simulink model "VDSE_2019b1"  (R2022b)
settings: Solver=ode5  StartTime=0.0  StopTime=T_simulation  FixedStep=simulation_step_time  RelTol=1e-3
values from neighbouring files (symbols this model uses):
  A = 2    [vehicle_parameters_script.m]
  bump_height = 0    [vehicle_parameters_script.m]
  bump_length = 0    [vehicle_parameters_script.m]
  bump_time = 0    [vehicle_parameters_script.m]
  cd = 0.35    [vehicle_parameters_script.m]
  cF = 5000    [vehicle_parameters_script.m]
  clF = -0.15    [vehicle_parameters_script.m]
  clR = -0.20    (= -0.2)    [vehicle_parameters_script.m]
  cp_FA = 30    [vehicle_parameters_script.m]
  cp_RA = 13    [vehicle_parameters_script.m]
  cR = 5000    [vehicle_parameters_script.m]
  ctF = tireF.VERTICAL_DAMPING    [vehicle_parameters_script.m]
  ctR = tireR.VERTICAL_DAMPING    [vehicle_parameters_script.m]
  enableDriverControl = 1    [vehicle_parameters_script.m]
  enableLongDynamics = 1    [vehicle_parameters_script.m]
  enablePowertrain = 1    [vehicle_parameters_script.m]
  g = 9.806    [vehicle_parameters_script.m]
  Gear_numbers = [1 2 3 4 5 6]    [vehicle_parameters_script.m]
  GR = [2.9 1.8 1.3 1 0.85 0.75]    [vehicle_parameters_script.m]
  hcog = 0.441    [vehicle_parameters_script.m]
  hpc = 0.0    (= 0)    [vehicle_parameters_script.m]
  hrcF = 0.3    [vehicle_parameters_script.m]
  hrcg = (hrcF*lR+hrcR*lF)/(lF+lR)    (= 0.25108)    [vehicle_parameters_script.m]
  hrcR = 0.2    [vehicle_parameters_script.m]
  huFcog = 0.32    [vehicle_parameters_script.m]
  huRcog = 0.32    [vehicle_parameters_script.m]
  i1 = 11.42    [vehicle_parameters_script.m]
  i2 = 3.727    [vehicle_parameters_script.m]
  initial_gear = 1    [vehicle_parameters_script.m]
  JwF = 2.45    [vehicle_parameters_script.m]
  JwR = 2.45    [vehicle_parameters_script.m]
  Jx = 4.12    [vehicle_parameters_script.m]
  Jy = 109.16    [vehicle_parameters_script.m]
  Jz = 105.13    [vehicle_parameters_script.m]
  kF = 40000    [vehicle_parameters_script.m]
  kR = 35000    [vehicle_parameters_script.m]
  kRF = 0    [vehicle_parameters_script.m]
  kRR = 0    [vehicle_parameters_script.m]
  ktF = tireF.VERTICAL_STIFFNESS    [vehicle_parameters_script.m]
  ktR = tireR.VERTICAL_STIFFNESS    [vehicle_parameters_script.m]
  lF = 1.223    [vehicle_parameters_script.m]
  lR = l-lF    (= 1.277)    [vehicle_parameters_script.m]
  m = 340    [vehicle_parameters_script.m]
  max_pressure = 1000    [vehicle_parameters_script.m]
  maxrpm = 4000    [vehicle_parameters_script.m]
  mF = 45    [vehicle_parameters_script.m]
  minrpm = 1500    [vehicle_parameters_script.m]
  mR = 50    [vehicle_parameters_script.m]
  output_samping_time = 0.001    [vehicle_parameters_script.m]
  phi0 = 0    [vehicle_parameters_script.m]
  phi_dot0 = 0    [vehicle_parameters_script.m]
  psi0 = 0    [vehicle_parameters_script.m]
  psi_dot0 = 0    [vehicle_parameters_script.m]
  RearRatio = 1    [vehicle_parameters_script.m]
  requested_speed = 120/3.6    (= 33.3333333333)    [vehicle_parameters_script.m]
  rF = tireF.UNLOADED_RADIUS    [vehicle_parameters_script.m]
  rho = 1.2    [vehicle_parameters_script.m]
  rR = tireR.UNLOADED_RADIUS    [vehicle_parameters_script.m]
  steer_ratio = 13.25    [vehicle_parameters_script.m]
  TFL = 0    [vehicle_parameters_script.m]
  TFR = 0    [vehicle_parameters_script.m]
  theta0 = 0    [vehicle_parameters_script.m]
  theta_dot0 = 0    [vehicle_parameters_script.m]
  TRL = 0    [vehicle_parameters_script.m]
  TRR = 0    [vehicle_parameters_script.m]
  Vx0 = 0.01/3.6    (= 0.00277777777778)    [vehicle_parameters_script.m]
  Vy0 = 0    [vehicle_parameters_script.m]
  Vz0 = 0    [vehicle_parameters_script.m]
  wF = 1.578    [vehicle_parameters_script.m]
  wR = 1.544    [vehicle_parameters_script.m]
  x0 = 0    [vehicle_parameters_script.m]
  xcog_overall = (2*mR*xR+2*xF*mF+m*xs)/(m+2*mF+2*mR)    (= 1.25626415094)    [vehicle_parameters_script.m]
  y0 = 0    [vehicle_parameters_script.m]
  z0 = 0    [vehicle_parameters_script.m]
  zFL0 = 0    [vehicle_parameters_script.m]
  zFL_dot0 = 0    [vehicle_parameters_script.m]
  zFR0 = 0    [vehicle_parameters_script.m]
  zFR_dot0 = 0    [vehicle_parameters_script.m]
  zRL0 = 0    [vehicle_parameters_script.m]
  zRL_dot0 = 0    [vehicle_parameters_script.m]
  zRR0 = 0    [vehicle_parameters_script.m]
  zRR_dot0 = 0    [vehicle_parameters_script.m]
undefined symbols (not defined in the file or in its folder): Bxf, Bxr, Byf, Byr, Cxf, Cxr, Cyf, Cyr, DiscIntNeverNeededParam, Dxf, Dxr, Dyf, Dyr, exf, exr, eyf, eyr, FNOMINf, FNOMINr, Ldwf, Ldwr, PCX1f, PCX1r, PCY1f, PCY1r, PDX1f, PDX1r, PDX2f, PDX2r, PDY1f, PDY1r, PDY2f, PDY2r, PDY3f, PDY3r, PEX1f, PEX1r, PEX2f, PEX2r, PEX3f, PEX3r, PEX4f, PEX4r, PEY1f, PEY1r, PEY2f, PEY2r, PEY3f, PEY3r, PEY4f, PEY4r, PHX1f, PHX1r, PHX2f, PHX2r, PHY1f, PHY1r, PHY2f, PHY2r, PHY3f ... (+147)
libraries: simulink x55, mfeval_LIB x4, slpidlib x1
(part 3 of 7)

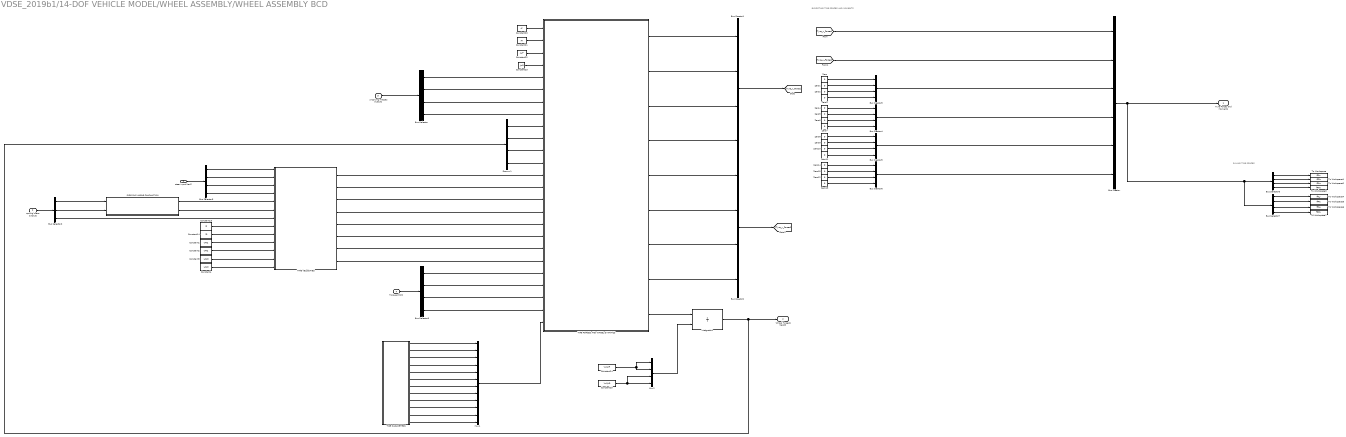
== system VDSE_2019b1/14-DOF VEHICLE MODEL/WHEEL ASSEMBLY/WHEEL ASSEMBLY BCD ==
  note: EXPORTING TIRE FORCES AND MOMENTS
  note: SAVING TIRE FORCES
  steer input [rad] : Inport
  sprung mass outputs : Inport  Port=2
  unsprung masses outputs : Inport  Port=3
  Torques [Nm] : Inport  Port=4
  Bus Creator : BusCreator  Inputs=6
  Bus Creator{1..6} (6 alike) : BusCreator  Inputs=4
  Bus Selector : BusSelector  OutputSignals=Unsprung masses z Forces [N].FLz_Overall [N],Unsprung masses z Forces [N].FRz_Overall [N],Unsprung masses z Forces [N].RLz_Overall [N],Unsprung masses z Forces [N].RRz_Overall [N]
  Bus Selector2 : BusSelector  OutputSignals=Longitudinal Dynamics.Vx [m/s],Lateral Dynamics.Vy [m/s],Yaw dynamics.psi_dot [rad/s]
  Bus Selector3 : BusSelector  OutputSignals=Steering.deltaFL [rad],Steering.deltaFR [rad],Steering.deltaRL [rad],Steering.deltaRR [rad]
  Bus Selector5 : BusSelector  OutputSignals=TFL [Nm],TFR [Nm],TRL [Nm],TRR [Nm]
  Bus Selector6 : BusSelector  OutputSignals=Tyre x Forces [N].fFLx [N],Tyre x Forces [N].fFRx [N],Tyre x Forces [N].fRLx [N],Tyre x Forces [N].fRRx [N]
  Bus Selector7 : BusSelector  OutputSignals=Tyre y Forces [N].fFLy [N],Tyre y Forces [N].fFRy [N],Tyre y Forces [N].fRLy [N],Tyre y Forces [N].fRRy [N]
  Constant1 : Constant  Value=wF/2
  Constant13 : Constant  Value=lF
  Constant14 : Constant  Value=lR
  Constant2 : Constant  Value=wF/2
  Constant20 : Constant  Value=rF
  Constant21 : Constant  Value=rR
  Constant22 : Constant  Value=JwF
  Constant23 : Constant  Value=JwR
  Constant24 : Constant  Value=Vx0/rF
  Constant25 : Constant  Value=Vx0/rR
  Constant3 : Constant  Value=wR/2
  Constant4 : Constant  Value=wR/2
  Demux1 : Demux
  Integrator1 : Integrator  InitialConditionSource=external
  Mux1 : Mux  Inputs=12
  Mux2 : Mux
  SIDE SLIP ANGLE CALCULATION : Subsystem
  TIRE FORCES AND WHEEL DYNAMICS : MATLAB Function  TreatAsAtomicUnit=on
  TIRE PARAMETERS : Subsystem
  TIRE VELOCITIES : MATLAB Function  TreatAsAtomicUnit=on
  To Workspace : ToWorkspace  VariableName=fFLx  SaveFormat=Timeseries  SampleTime=-1
  To Workspace1 : ToWorkspace  VariableName=fFRx  SaveFormat=Timeseries  SampleTime=-1
  To Workspace2 : ToWorkspace  VariableName=fRLx  SaveFormat=Timeseries  SampleTime=-1
  To Workspace3 : ToWorkspace  VariableName=fRRx  SaveFormat=Timeseries  SampleTime=-1
  To Workspace4 : ToWorkspace  VariableName=fFLy  SaveFormat=Timeseries  SampleTime=-1
  To Workspace5 : ToWorkspace  VariableName=fFRy  SaveFormat=Timeseries  SampleTime=-1
  To Workspace6 : ToWorkspace  VariableName=fRLy  SaveFormat=Timeseries  SampleTime=-1
  To Workspace7 : ToWorkspace  VariableName=fRRy  SaveFormat=Timeseries  SampleTime=-1
  Zero{,1..15} (16 alike) : Constant  Value=0  OutDataTypeStr=Inherit: Inherit via back propagation
  Tyre Forces and Moments : Outport
  Wheel Speeds [rad/s] : Outport  Port=2
  wires:
  Bus Selector7/4 -> To Workspace7/1  "<fRRy [N]>"
  Bus Selector7/3 -> To Workspace6/1  "<fRLy [N]>"
  Bus Selector7/2 -> To Workspace5/1  "<fFRy [N]>"
  Bus Selector7/1 -> To Workspace4/1  "<fFLy [N]>"
  Bus Selector6/4 -> To Workspace3/1  "<fRRx [N]>"
  Bus Selector6/3 -> To Workspace2/1  "<fRLx [N]>"
  Bus Selector6/2 -> To Workspace1/1  "<fFRx [N]>"
  Bus Selector6/1 -> To Workspace/1  "<fFLx [N]>"
  Torques [Nm]/1 -> Bus Selector5/1
  Bus Creator/1 -> Tyre Forces and Moments/1, Bus Selector6/1, Bus Selector7/1
  steer input [rad]/1 -> Bus Selector3/1
  Bus Selector3/3 -> TIRE VELOCITIES/3(deltaRL)  "<deltaRL [rad]>"
  Bus Selector3/1 -> TIRE VELOCITIES/1(deltaFL)  "<deltaFL [rad]>"
  Bus Selector3/4 -> TIRE VELOCITIES/4(deltaRR)  "<deltaRR [rad]>"
  Bus Selector3/2 -> TIRE VELOCITIES/2(deltaFR)  "<deltaFR [rad]>"
  sprung mass outputs/1 -> Bus Selector2/1
  Bus Selector2/3 -> TIRE VELOCITIES/7(psidot)  "<psi_dot [rad/s]>"
  Bus Selector2/2 -> SIDE SLIP ANGLE CALCULATION/2(Vy [m/s])  "<Vy [m/s]>"
  Bus Selector2/1 -> SIDE SLIP ANGLE CALCULATION/1(Vx [m/s])  "<Vx [m/s]>"
  unsprung masses outputs/1 -> Bus Selector/1
  Bus Selector/2 -> TIRE FORCES AND WHEEL DYNAMICS/6(fFRz)  "<FRz_Overall [N]>"
  Bus Selector/3 -> TIRE FORCES AND WHEEL DYNAMICS/7(fRLz)  "<RLz_Overall [N]>"
  Bus Selector/4 -> TIRE FORCES AND WHEEL DYNAMICS/8(fRRz)  "<RRz_Overall [N]>"
  Bus Selector/1 -> TIRE FORCES AND WHEEL DYNAMICS/5(fFLz)  "<FLz_Overall [N]>"
  SIDE SLIP ANGLE CALCULATION/1(V [m/s]) -> TIRE VELOCITIES/5(V)  "V"
  SIDE SLIP ANGLE CALCULATION/2(beta [rad]) -> TIRE VELOCITIES/6(beta)  "beta"
  TIRE VELOCITIES/6(VRLy) -> TIRE FORCES AND WHEEL DYNAMICS/18(VRLy)  "VRLy"
  TIRE VELOCITIES/3(VFRx) -> TIRE FORCES AND WHEEL DYNAMICS/15(VFRx)  "VFRx"
  Constant3/1 -> TIRE VELOCITIES/12(wRL)
  TIRE VELOCITIES/5(VRLx) -> TIRE FORCES AND WHEEL DYNAMICS/17(VRLx)  "VRLx"
  Constant2/1 -> TIRE VELOCITIES/11(wFR)
  Constant14/1 -> TIRE VELOCITIES/9(lR)
  Constant1/1 -> TIRE VELOCITIES/10(wFL)
  Constant13/1 -> TIRE VELOCITIES/8(lF)
  Constant4/1 -> TIRE VELOCITIES/13(wRR)
  TIRE VELOCITIES/4(VFRy) -> TIRE FORCES AND WHEEL DYNAMICS/16(VFRy)  "VFRy"
  TIRE VELOCITIES/1(VFLx) -> TIRE FORCES AND WHEEL DYNAMICS/13(VFLx)  "VFLx"
  TIRE VELOCITIES/2(VFLy) -> TIRE FORCES AND WHEEL DYNAMICS/14(VFLy)  "VFLy"
  TIRE PARAMETERS/7(Byf) -> Mux1/7
  TIRE PARAMETERS/6(Dxr) -> Mux1/6
  TIRE PARAMETERS/12(Dyr) -> Mux1/12
  TIRE PARAMETERS/2(Cxf) -> Mux1/2
  Mux1/1 -> TIRE FORCES AND WHEEL DYNAMICS/25(TireParams)
  TIRE PARAMETERS/8(Cyf) -> Mux1/8
  TIRE PARAMETERS/9(Dyf) -> Mux1/9
  TIRE PARAMETERS/5(Cxr) -> Mux1/5
  TIRE PARAMETERS/3(Dxf) -> Mux1/3
  TIRE PARAMETERS/11(Cyr) -> Mux1/11
  TIRE PARAMETERS/10(Byr) -> Mux1/10
  TIRE PARAMETERS/4(Bxr) -> Mux1/4
  TIRE PARAMETERS/1(Bxf) -> Mux1/1
  Constant20/1 -> TIRE FORCES AND WHEEL DYNAMICS/1(rF)
  Constant22/1 -> TIRE FORCES AND WHEEL DYNAMICS/3(JwF)
  Constant23/1 -> TIRE FORCES AND WHEEL DYNAMICS/4(JwR)
  Constant21/1 -> TIRE FORCES AND WHEEL DYNAMICS/2(rR)
  Constant24/1 -> Mux2/2, Mux2/1
  Mux2/1 -> Integrator1/2
  Constant25/1 -> Mux2/3, Mux2/4
  TIRE FORCES AND WHEEL DYNAMICS/9(omega_dot) -> Integrator1/1  "omegas_dot [rad/s^2]"
  Demux1/1 -> TIRE FORCES AND WHEEL DYNAMICS/9(omegaFL)
  Demux1/2 -> TIRE FORCES AND WHEEL DYNAMICS/10(omegaFR)
  Demux1/3 -> TIRE FORCES AND WHEEL DYNAMICS/11(omegaRL)
  Demux1/4 -> TIRE FORCES AND WHEEL DYNAMICS/12(omegaRR)
  Integrator1/1 -> Demux1/1, Wheel Speeds [rad/s]/1  "omega [rad/s]"
  TIRE VELOCITIES/7(VRRx) -> TIRE FORCES AND WHEEL DYNAMICS/19(VRRx)  "VRRx"
  TIRE VELOCITIES/8(VRRy) -> TIRE FORCES AND WHEEL DYNAMICS/20(VRRy)  "VRRy"
  TIRE FORCES AND WHEEL DYNAMICS/6(fFRy) -> Bus Creator2/2  "fFRy [N]"
  TIRE FORCES AND WHEEL DYNAMICS/3(fRLx) -> Bus Creator1/3  "fRLx [N]"
  TIRE FORCES AND WHEEL DYNAMICS/4(fRRx) -> Bus Creator1/4  "fRRx [N]"
  Bus Creator1/1 -> [Tyre_x_Forces]  "Tyre x Forces [N]"
  TIRE FORCES AND WHEEL DYNAMICS/5(fFLy) -> Bus Creator2/1  "fFLy [N]"
  TIRE FORCES AND WHEEL DYNAMICS/7(fRLy) -> Bus Creator2/3  "fRLy [N]"
  TIRE FORCES AND WHEEL DYNAMICS/8(fRRy) -> Bus Creator2/4  "fRRy [N]"
  Bus Creator2/1 -> [Tyre_y_Forces]  "Tyre y Forces [N]"
  Zero6/1 -> Bus Creator4/3  "mRLx [Nm]"
  Zero3/1 -> Bus Creator3/4  "fRRz [N]"
  Zero5/1 -> Bus Creator4/2  "mFRx [Nm]"
  Zero7/1 -> Bus Creator4/4  "mRRx [Nm]"
  Zero1/1 -> Bus Creator3/2  "fFRz [N]"
  Zero4/1 -> Bus Creator4/1  "mFLx [Nm]"
  Zero2/1 -> Bus Creator3/3  "fRLz [N]"
  Zero/1 -> Bus Creator3/1  "fFLz [N]"
  Zero13/1 -> Bus Creator6/4  "mRRz [Nm]"
  Zero12/1 -> Bus Creator6/3  "mRLz [Nm]"
  Zero15/1 -> Bus Creator6/2  "mFRz [Nm]"
  Zero14/1 -> Bus Creator6/1  "mFLz [Nm]"
  TIRE FORCES AND WHEEL DYNAMICS/1(fFLx) -> Bus Creator1/1  "fFLx [N]"
  TIRE FORCES AND WHEEL DYNAMICS/2(fFRx) -> Bus Creator1/2  "fFRx [N]"
  [Tyre_x_Forces] -> Bus Creator/1  "Tyre x Forces [N]"
  [Tyre_y_Forces] -> Bus Creator/2  "Tyre y Forces [N]"
  Bus Creator3/1 -> Bus Creator/3  "Tyre z Forces [N]"
  Bus Creator4/1 -> Bus Creator/4  "Tyre Mx Moments [Nm]"
  Bus Creator5/1 -> Bus Creator/5  "Tyre My Moments [Nm]"
  Bus Creator6/1 -> Bus Creator/6  "Tyre Mz Moments [Nm]"
  Zero8/1 -> Bus Creator5/1  "mFLy [Nm]"
  Zero9/1 -> Bus Creator5/2  "mFRy [Nm]"
  Zero10/1 -> Bus Creator5/3  "mRLy [Nm]"
  Zero11/1 -> Bus Creator5/4  "mRRy [Nm]"
  Bus Selector5/1 -> TIRE FORCES AND WHEEL DYNAMICS/21(TFL)  "<TFL [Nm]>"
  Bus Selector5/2 -> TIRE FORCES AND WHEEL DYNAMICS/22(TFR)  "<TFR [Nm]>"
  Bus Selector5/3 -> TIRE FORCES AND WHEEL DYNAMICS/23(TRL)  "<TRL [Nm]>"
  Bus Selector5/4 -> TIRE FORCES AND WHEEL DYNAMICS/24(TRR)  "<TRR [Nm]>"

== system VDSE_2019b1/14-DOF VEHICLE MODEL/WHEEL ASSEMBLY/WHEEL ASSEMBLY MFEVAL ==
  note: EXPORT TIRE FORCES AND MOMENTS
  note: Wheel Dynamics:
      |
      | J_w∙ω_FR_dot=T_FR- F_FR∙r_w
      | J_w∙ω_FL_dot=T_FL- F_FL∙r_w
      | J_w∙ω_RL_dot= T_RL- F_RL∙r_w
      | J_w∙ω_RR_dot= T_RR- F_RR∙r_w
  note: SAVING TIRE FORCES
  steer input [rad] : Inport
  sprung mass outputs : Inport  Port=2
  unsprung masses outputs : Inport  Port=3
  Torques [Nm] : Inport  Port=4
  Bus Creator : BusCreator  Inputs=6
  Bus Selector : BusSelector  OutputSignals=Unsprung masses z Forces [N].FLz_Overall [N],Unsprung masses z Forces [N].FRz_Overall [N],Unsprung masses z Forces [N].RLz_Overall [N],Unsprung masses z Forces [N].RRz_Overall [N]
  Bus Selector1 : BusSelector  OutputSignals=fFLx [N],fFRx [N],fRLx [N],fRRx [N]
  Bus Selector2 : BusSelector  OutputSignals=Longitudinal Dynamics.Vx [m/s],Lateral Dynamics.Vy [m/s],Yaw dynamics.psi_dot [rad/s]
  Bus Selector3 : BusSelector  OutputSignals=Steering.deltaFL [rad],Steering.deltaFR [rad],Steering.deltaRL [rad],Steering.deltaRR [rad]
  Bus Selector5 : BusSelector  OutputSignals=TFL [Nm],TFR [Nm],TRL [Nm],TRR [Nm]
  Bus Selector6 : BusSelector  OutputSignals=Tyre x Forces [N].fFLx [N],Tyre x Forces [N].fFRx [N],Tyre x Forces [N].fRLx [N],Tyre x Forces [N].fRRx [N]
  Bus Selector7 : BusSelector  OutputSignals=Tyre y Forces [N].fFLy [N],Tyre y Forces [N].fFRy [N],Tyre y Forces [N].fRLy [N],Tyre y Forces [N].fRRy [N]
  Constant : Constant  Value=Vx0/rF
  Constant1 : Constant  Value=wF/2
  Constant13 : Constant  Value=lF
  Constant14 : Constant  Value=lR
  Constant2 : Constant  Value=wF/2
  Constant3 : Constant  Value=wR/2
  Constant4 : Constant  Value=wR/2
  Constant5 : Constant  Value=rF
  Constant6 : Constant  Value=rR
  Constant7 : Constant  Value=Vx0/rR
  Constant8 : Constant  Value=JwF
  Constant9 : Constant  Value=JwR
  Demux : Demux
  Integrator2 : Integrator  InitialConditionSource=external
  Mux : Mux
  SIDE SLIP ANGLE CALCULATION : Subsystem
  Saturation : Saturate  UpperLimit=5000  LowerLimit=-5000
  TIRE CALCULATION : Subsystem
  TIRE VELOCITIES : MATLAB Function  TreatAsAtomicUnit=on
  To Workspace : ToWorkspace  VariableName=fFLx  SaveFormat=Timeseries  SampleTime=-1
  To Workspace1 : ToWorkspace  VariableName=fFRx  SaveFormat=Timeseries  SampleTime=-1
  To Workspace2 : ToWorkspace  VariableName=fRLx  SaveFormat=Timeseries  SampleTime=-1
  To Workspace3 : ToWorkspace  VariableName=fRRx  SaveFormat=Timeseries  SampleTime=-1
  To Workspace4 : ToWorkspace  VariableName=fFLy  SaveFormat=Timeseries  SampleTime=-1
  To Workspace5 : ToWorkspace  VariableName=fFRy  SaveFormat=Timeseries  SampleTime=-1
  To Workspace6 : ToWorkspace  VariableName=fRLy  SaveFormat=Timeseries  SampleTime=-1
  To Workspace7 : ToWorkspace  VariableName=fRRy  SaveFormat=Timeseries  SampleTime=-1
  WHEEL DYNAMICS : MATLAB Function  TreatAsAtomicUnit=on
  Tyre Forces and Moments : Outport
  Wheel Speeds [rad/s] : Outport  Port=2
  wires:
  TIRE CALCULATION/4(Tyre Mx Moments [Nm]) -> Bus Creator/4  "Tyre Mx Moments [Nm]"
  Bus Selector7/4 -> To Workspace7/1  "<fRRy [N]>"
  Bus Selector7/3 -> To Workspace6/1  "<fRLy [N]>"
  Bus Selector7/2 -> To Workspace5/1  "<fFRy [N]>"
  Bus Selector7/1 -> To Workspace4/1  "<fFLy [N]>"
  Bus Selector6/4 -> To Workspace3/1  "<fRRx [N]>"
  Bus Selector6/3 -> To Workspace2/1  "<fRLx [N]>"
  Bus Selector6/2 -> To Workspace1/1  "<fFRx [N]>"
  Bus Selector6/1 -> To Workspace/1  "<fFLx [N]>"
  Torques [Nm]/1 -> Bus Selector5/1
  Bus Creator/1 -> Bus Selector6/1, Bus Selector7/1, Tyre Forces and Moments/1
  steer input [rad]/1 -> Bus Selector3/1
  Bus Selector3/3 -> TIRE VELOCITIES/3(deltaRL)  "<deltaRL [rad]>"
  Bus Selector3/1 -> TIRE VELOCITIES/1(deltaFL)  "<deltaFL [rad]>"
  Bus Selector3/4 -> TIRE VELOCITIES/4(deltaRR)  "<deltaRR [rad]>"
  Bus Selector3/2 -> TIRE VELOCITIES/2(deltaFR)  "<deltaFR [rad]>"
  sprung mass outputs/1 -> Bus Selector2/1
  Bus Selector2/3 -> TIRE VELOCITIES/7(psidot)  "<psi_dot [rad/s]>"
  unsprung masses outputs/1 -> Bus Selector/1
  Bus Selector/2 -> TIRE CALCULATION/2(fFRz [N])  "<FRz_Overall [N]>"
  Bus Selector/3 -> TIRE CALCULATION/3(fRLz [N])  "<RLz_Overall [N]>"
  Bus Selector/4 -> TIRE CALCULATION/4(fRRz [N])  "<RRz_Overall [N]>"
  Bus Selector/1 -> TIRE CALCULATION/1(fFLz [N])  "<FLz_Overall [N]>"
  SIDE SLIP ANGLE CALCULATION/1(V [m/s]) -> TIRE VELOCITIES/5(V)  "V"
  SIDE SLIP ANGLE CALCULATION/2(beta [rad]) -> TIRE VELOCITIES/6(beta)  "beta"
  TIRE VELOCITIES/8(VRRy) -> TIRE CALCULATION/16(VRRy [m/s])  "VRRy"
  TIRE VELOCITIES/7(VRRx) -> TIRE CALCULATION/15(VRRx [m/s])  "VRRx"
  TIRE VELOCITIES/6(VRLy) -> TIRE CALCULATION/14(VRLy [m/s])  "VRLy"
  TIRE VELOCITIES/3(VFRx) -> TIRE CALCULATION/11(VFRx [m/s])  "VFRx"
  Bus Selector1/1 -> WHEEL DYNAMICS/5(fFLx)  "<fFLx [N]>"
  Constant9/1 -> WHEEL DYNAMICS/4(JwR)
  Constant3/1 -> TIRE VELOCITIES/12(wRL)
  TIRE VELOCITIES/5(VRLx) -> TIRE CALCULATION/13(VRLx [m/s])  "VRLx"
  Constant2/1 -> TIRE VELOCITIES/11(wFR)
  Demux/4 -> TIRE CALCULATION/8(omegaRR [rad/s])  "omegaRR [rad/s]"
  Constant/1 -> Mux/1, Mux/2
  Demux/3 -> TIRE CALCULATION/7(omegaRL [rad/s])  "omegaRL [rad/s]"
  Demux/1 -> TIRE CALCULATION/5(omegaFL [rad/s])  "omegaFL [rad/s]"
  WHEEL DYNAMICS/1(omega_dot) -> Saturation/1  "omegas_dot [rad/s^2]"
  Constant14/1 -> TIRE VELOCITIES/9(lR)
  Constant8/1 -> WHEEL DYNAMICS/3(JwF)
  Constant1/1 -> TIRE VELOCITIES/10(wFL)
  Mux/1 -> Integrator2/2
  Constant5/1 -> WHEEL DYNAMICS/1(rF)
  Constant13/1 -> TIRE VELOCITIES/8(lF)
  Integrator2/1 -> Wheel Speeds [rad/s]/1, Demux/1  "omega [rad/s]"
  Bus Selector1/2 -> WHEEL DYNAMICS/6(fFRx)  "<fFRx [N]>"
  Constant4/1 -> TIRE VELOCITIES/13(wRR)
  Bus Selector1/3 -> WHEEL DYNAMICS/7(fRLx)  "<fRLx [N]>"
  TIRE VELOCITIES/4(VFRy) -> TIRE CALCULATION/12(VFRy [m/s])  "VFRy"
  TIRE VELOCITIES/1(VFLx) -> TIRE CALCULATION/9(VFLx [m/s])  "VFLx"
  Constant6/1 -> WHEEL DYNAMICS/2(rR)
  Demux/2 -> TIRE CALCULATION/6(omegaFR [rad/s])  "omegaFR [rad/s]"
  Constant7/1 -> Mux/4, Mux/3
  Bus Selector1/4 -> WHEEL DYNAMICS/8(fRRx)  "<fRRx [N]>"
  TIRE VELOCITIES/2(VFLy) -> TIRE CALCULATION/10(VFLy [m/s])  "VFLy"
  TIRE CALCULATION/1(Tyre x Forces [N]) -> Bus Creator/1, Bus Selector1/1  "Tyre x Forces [N]"
  TIRE CALCULATION/2(Tyre y Forces [N]) -> Bus Creator/2  "Tyre y Forces [N]"
  TIRE CALCULATION/6(Tyre Mz Moments [Nm]) -> Bus Creator/6  "Tyre Mz Moments [Nm]"
  TIRE CALCULATION/3(Tyre z Forces [N]) -> Bus Creator/3  "Tyre z Forces [N]"
  TIRE CALCULATION/5(Tyre My Moments [Nm]) -> Bus Creator/5  "Tyre My Moments [Nm]"
  Bus Selector2/2 -> SIDE SLIP ANGLE CALCULATION/2(Vy [m/s])  "<Vy [m/s]>"
  Bus Selector2/1 -> SIDE SLIP ANGLE CALCULATION/1(Vx [m/s])  "<Vx [m/s]>"
  Bus Selector5/1 -> WHEEL DYNAMICS/9(TFL)  "<TFL [Nm]>"
  Bus Selector5/2 -> WHEEL DYNAMICS/10(TFR)  "<TFR [Nm]>"
  Bus Selector5/3 -> WHEEL DYNAMICS/11(TRL)  "<TRL [Nm]>"
  Bus Selector5/4 -> WHEEL DYNAMICS/12(TRR)  "<TRR [Nm]>"
  Saturation/1 -> Integrator2/1

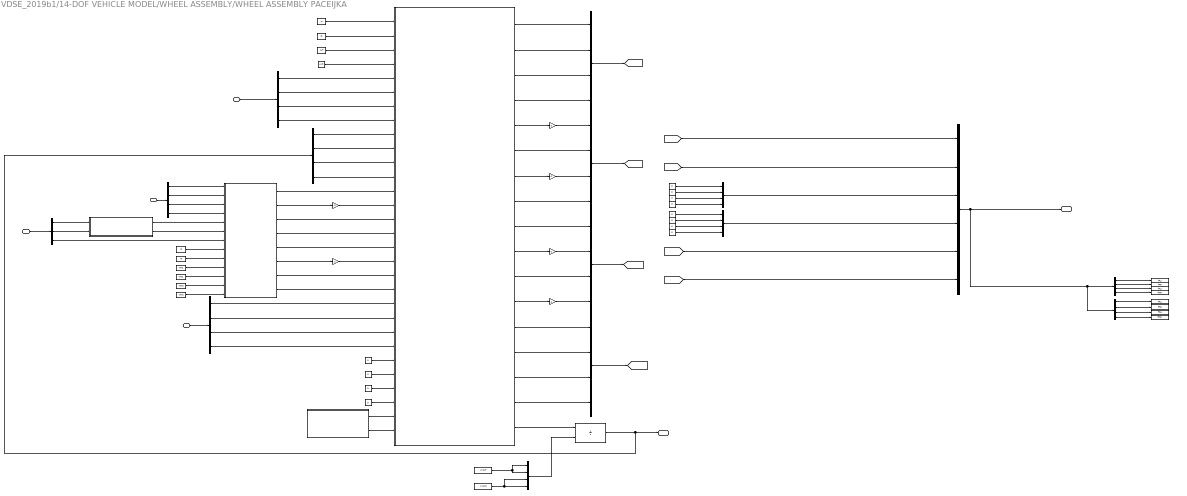
== system VDSE_2019b1/14-DOF VEHICLE MODEL/WHEEL ASSEMBLY/WHEEL ASSEMBLY PACEIJKA ==
  note: EXPORTING TIRE FORCES AND MOMENTS
  note: SAVING TIRE FORCES
  steer input [rad] : Inport
  sprung mass outputs : Inport  Port=2
  unsprung masses outputs : Inport  Port=3
  Torques [Nm] : Inport  Port=4
  Bus Creator : BusCreator  Inputs=6
  Bus Creator{1..4,7..8} (6 alike) : BusCreator  Inputs=4
  Bus Selector : BusSelector  OutputSignals=Unsprung masses z Forces [N].FLz_Overall [N],Unsprung masses z Forces [N].FRz_Overall [N],Unsprung masses z Forces [N].RLz_Overall [N],Unsprung masses z Forces [N].RRz_Overall [N]
  Bus Selector2 : BusSelector  OutputSignals=Longitudinal Dynamics.Vx [m/s],Lateral Dynamics.Vy [m/s],Yaw dynamics.psi_dot [rad/s]
  Bus Selector3 : BusSelector  OutputSignals=Steering.deltaFL [rad],Steering.deltaFR [rad],Steering.deltaRL [rad],Steering.deltaRR [rad]
  Bus Selector5 : BusSelector  OutputSignals=TFL [Nm],TFR [Nm],TRL [Nm],TRR [Nm]
  Bus Selector6 : BusSelector  OutputSignals=Tyre x Forces [N].fFLx [N],Tyre x Forces [N].fFRx [N],Tyre x Forces [N].fRLx [N],Tyre x Forces [N].fRRx [N]
  Bus Selector7 : BusSelector  OutputSignals=Tyre y Forces [N].fFLy [N],Tyre y Forces [N].fFRy [N],Tyre y Forces [N].fRLy [N],Tyre y Forces [N].fRRy [N]
  Constant{,26..28} (4 alike) : Constant  Value=0
  Constant1 : Constant  Value=wF/2
  Constant13 : Constant  Value=lF
  Constant14 : Constant  Value=lR
  Constant2 : Constant  Value=wF/2
  Constant20 : Constant  Value=rF
  Constant21 : Constant  Value=rR
  Constant22 : Constant  Value=JwF
  Constant23 : Constant  Value=JwR
  Constant24 : Constant  Value=Vx0/rF
  Constant25 : Constant  Value=Vx0/rR
  Constant3 : Constant  Value=wR/2
  Constant4 : Constant  Value=wR/2
  Demux1 : Demux
  Gain{,1..5} (6 alike) : Gain  Gain=-1
  Integrator1 : Integrator  InitialConditionSource=external
  Mux2 : Mux
  SIDE SLIP ANGLE CALCULATION : Subsystem
  TIRE FORCES AND WHEEL DYNAMICS : MATLAB Function  TreatAsAtomicUnit=on
  TIRE PARAMETERS : Subsystem
  TIRE VELOCITIES : MATLAB Function  TreatAsAtomicUnit=on
  To Workspace : ToWorkspace  VariableName=fFLx  SaveFormat=Timeseries  SampleTime=-1
  To Workspace1 : ToWorkspace  VariableName=fFRx  SaveFormat=Timeseries  SampleTime=-1
  To Workspace2 : ToWorkspace  VariableName=fRLx  SaveFormat=Timeseries  SampleTime=-1
  To Workspace3 : ToWorkspace  VariableName=fRRx  SaveFormat=Timeseries  SampleTime=-1
  To Workspace4 : ToWorkspace  VariableName=fFLy  SaveFormat=Timeseries  SampleTime=-1
  To Workspace5 : ToWorkspace  VariableName=fFRy  SaveFormat=Timeseries  SampleTime=-1
  To Workspace6 : ToWorkspace  VariableName=fRLy  SaveFormat=Timeseries  SampleTime=-1
  To Workspace7 : ToWorkspace  VariableName=fRRy  SaveFormat=Timeseries  SampleTime=-1
  Zero{,1..7} (8 alike) : Constant  Value=0  OutDataTypeStr=Inherit: Inherit via back propagation
  Tyre Forces and Moments : Outport
  Wheel Speeds [rad/s] : Outport  Port=2
  wires:
  Zero/1 -> Bus Creator3/1  "fFLz [N]"
  Zero2/1 -> Bus Creator3/3  "fRLz [N]"
  Zero4/1 -> Bus Creator4/1  "mFLx [Nm]"
  Zero1/1 -> Bus Creator3/2  "fFRz [N]"
  Zero7/1 -> Bus Creator4/4  "mRRx [Nm]"
  Zero5/1 -> Bus Creator4/2  "mFRx [Nm]"
  Zero3/1 -> Bus Creator3/4  "fRRz [N]"
  Zero6/1 -> Bus Creator4/3  "mRLx [Nm]"
  Bus Creator2/1 -> [Tyre_y_Forces]  "Tyre y Forces [N]"
  TIRE FORCES AND WHEEL DYNAMICS/7(fRLy) -> Gain2/1  "fRLy [N]"
  TIRE FORCES AND WHEEL DYNAMICS/5(fFLy) -> Gain3/1  "fFLy [N]"
  Bus Creator1/1 -> [Tyre_x_Forces]  "Tyre x Forces [N]"
  TIRE VELOCITIES/8(VRRy) -> TIRE FORCES AND WHEEL DYNAMICS/20(VRRy)  "VRRy"
  TIRE VELOCITIES/7(VRRx) -> TIRE FORCES AND WHEEL DYNAMICS/19(VRRx)  "VRRx"
  Integrator1/1 -> Wheel Speeds [rad/s]/1, Demux1/1  "omega [rad/s]"
  Demux1/4 -> TIRE FORCES AND WHEEL DYNAMICS/12(omegaRR)
  Demux1/3 -> TIRE FORCES AND WHEEL DYNAMICS/11(omegaRL)
  Demux1/2 -> TIRE FORCES AND WHEEL DYNAMICS/10(omegaFR)
  Demux1/1 -> TIRE FORCES AND WHEEL DYNAMICS/9(omegaFL)
  TIRE FORCES AND WHEEL DYNAMICS/17(omega_dot) -> Integrator1/1  "omegas_dot [rad/s^2]"
  Constant25/1 -> Mux2/4, Mux2/3
  Mux2/1 -> Integrator1/2
  Constant24/1 -> Mux2/1, Mux2/2
  Constant21/1 -> TIRE FORCES AND WHEEL DYNAMICS/2(rR)
  Constant23/1 -> TIRE FORCES AND WHEEL DYNAMICS/4(JwR)
  Constant22/1 -> TIRE FORCES AND WHEEL DYNAMICS/3(JwF)
  Constant20/1 -> TIRE FORCES AND WHEEL DYNAMICS/1(rF)
  TIRE VELOCITIES/2(VFLy) -> Gain/1  "VFLy"
  TIRE VELOCITIES/1(VFLx) -> TIRE FORCES AND WHEEL DYNAMICS/13(VFLx)  "VFLx"
  TIRE VELOCITIES/4(VFRy) -> TIRE FORCES AND WHEEL DYNAMICS/16(VFRy)  "VFRy"
  Constant4/1 -> TIRE VELOCITIES/13(wRR)
  Constant13/1 -> TIRE VELOCITIES/8(lF)
  Constant1/1 -> TIRE VELOCITIES/10(wFL)
  Constant14/1 -> TIRE VELOCITIES/9(lR)
  Constant2/1 -> TIRE VELOCITIES/11(wFR)
  TIRE VELOCITIES/5(VRLx) -> TIRE FORCES AND WHEEL DYNAMICS/17(VRLx)  "VRLx"
  Constant3/1 -> TIRE VELOCITIES/12(wRL)
  TIRE VELOCITIES/3(VFRx) -> TIRE FORCES AND WHEEL DYNAMICS/15(VFRx)  "VFRx"
  TIRE VELOCITIES/6(VRLy) -> Gain1/1  "VRLy"
  SIDE SLIP ANGLE CALCULATION/2(beta [rad]) -> TIRE VELOCITIES/6(beta)  "beta"
  SIDE SLIP ANGLE CALCULATION/1(V [m/s]) -> TIRE VELOCITIES/5(V)  "V"
  Bus Selector/1 -> TIRE FORCES AND WHEEL DYNAMICS/5(fFLz)  "<FLz_Overall [N]>"
  Bus Selector/4 -> TIRE FORCES AND WHEEL DYNAMICS/8(fRRz)  "<RRz_Overall [N]>"
  Bus Selector/3 -> TIRE FORCES AND WHEEL DYNAMICS/7(fRLz)  "<RLz_Overall [N]>"
  Bus Selector/2 -> TIRE FORCES AND WHEEL DYNAMICS/6(fFRz)  "<FRz_Overall [N]>"
  unsprung masses outputs/1 -> Bus Selector/1
  sprung mass outputs/1 -> Bus Selector2/1
  Bus Selector3/2 -> TIRE VELOCITIES/2(deltaFR)  "<deltaFR [rad]>"
  Bus Selector3/4 -> TIRE VELOCITIES/4(deltaRR)  "<deltaRR [rad]>"
  Bus Selector3/1 -> TIRE VELOCITIES/1(deltaFL)  "<deltaFL [rad]>"
  Bus Selector3/3 -> TIRE VELOCITIES/3(deltaRL)  "<deltaRL [rad]>"
  steer input [rad]/1 -> Bus Selector3/1
  Bus Creator/1 -> Bus Selector7/1, Bus Selector6/1, Tyre Forces and Moments/1
  Torques [Nm]/1 -> Bus Selector5/1
  Bus Selector6/1 -> To Workspace/1  "<fFLx [N]>"
  Bus Selector6/2 -> To Workspace1/1  "<fFRx [N]>"
  Bus Selector6/3 -> To Workspace2/1  "<fRLx [N]>"
  Bus Selector6/4 -> To Workspace3/1  "<fRRx [N]>"
  Bus Selector7/1 -> To Workspace4/1  "<fFLy [N]>"
  Bus Selector7/2 -> To Workspace5/1  "<fFRy [N]>"
  Bus Selector7/3 -> To Workspace6/1  "<fRLy [N]>"
  Bus Selector7/4 -> To Workspace7/1  "<fRRy [N]>"
  [Tyre_y_Moments] -> Bus Creator/5  "Tyre My Moments [Nm]"
  Constant/1 -> TIRE FORCES AND WHEEL DYNAMICS/25(gammaFL)
  Constant26/1 -> TIRE FORCES AND WHEEL DYNAMICS/26(gammaFR)
  Constant27/1 -> TIRE FORCES AND WHEEL DYNAMICS/27(gammaRL)
  Constant28/1 -> TIRE FORCES AND WHEEL DYNAMICS/28(gammaRR)
  TIRE PARAMETERS/1(Tire Parameters Front Axle) -> TIRE FORCES AND WHEEL DYNAMICS/29(TireParams_front)
  TIRE PARAMETERS/2(Tire Parameters Rear Axle) -> TIRE FORCES AND WHEEL DYNAMICS/30(TireParams_rear)
  Gain/1 -> TIRE FORCES AND WHEEL DYNAMICS/14(VFLy)  "VFLy"
  Gain1/1 -> TIRE FORCES AND WHEEL DYNAMICS/18(VRLy)  "VRLy"
  TIRE FORCES AND WHEEL DYNAMICS/1(fFLx) -> Bus Creator1/1  "fFLx [N]"
  TIRE FORCES AND WHEEL DYNAMICS/2(fFRx) -> Bus Creator1/2  "fFRx [N]"
  TIRE FORCES AND WHEEL DYNAMICS/3(fRLx) -> Bus Creator1/3  "fRLx [N]"
  TIRE FORCES AND WHEEL DYNAMICS/4(fRRx) -> Bus Creator1/4  "fRRx [N]"
  Gain3/1 -> Bus Creator2/1  "fFLy [N]"
  TIRE FORCES AND WHEEL DYNAMICS/6(fFRy) -> Bus Creator2/2  "fFRy [N]"
  Gain2/1 -> Bus Creator2/3  "fRLy [N]"
  TIRE FORCES AND WHEEL DYNAMICS/8(fRRy) -> Bus Creator2/4  "fRRy [N]"
  [Tyre_x_Forces] -> Bus Creator/1  "Tyre x Forces [N]"
  [Tyre_y_Forces] -> Bus Creator/2  "Tyre y Forces [N]"
  Bus Creator3/1 -> Bus Creator/3  "Tyre z Forces [N]"
  Bus Creator4/1 -> Bus Creator/4  "Tyre Mx Moments [Nm]"
  [Tyre_z_Moments] -> Bus Creator/6  "Tyre Mz Moments [Nm]"
  TIRE FORCES AND WHEEL DYNAMICS/9(mFLz) -> Bus Creator7/1  "mFLz [Nm]"
  TIRE FORCES AND WHEEL DYNAMICS/10(mFRz) -> Gain4/1  "mFRz [Nm]"
  Gain4/1 -> Bus Creator7/2  "mFRz [Nm]"
  TIRE FORCES AND WHEEL DYNAMICS/11(mRLz) -> Bus Creator7/3  "mRLz [Nm]"
  TIRE FORCES AND WHEEL DYNAMICS/12(mRRz) -> Gain5/1  "mRRz [Nm]"
  Gain5/1 -> Bus Creator7/4  "mRRz [Nm]"
  TIRE FORCES AND WHEEL DYNAMICS/13(mFLy) -> Bus Creator8/1  "mFLy [Nm]"
  TIRE FORCES AND WHEEL DYNAMICS/14(mFRy) -> Bus Creator8/2  "mFRy [Nm]"
  TIRE FORCES AND WHEEL DYNAMICS/15(mRLy) -> Bus Creator8/3  "mRLy [Nm]"
  TIRE FORCES AND WHEEL DYNAMICS/16(mRRy) -> Bus Creator8/4  "mRRy [Nm]"
  Bus Creator7/1 -> [Tyre_z_Moments]  "Tyre Mz Moments [Nm]"
  Bus Creator8/1 -> [Tyre_y_Moments]  "Tyre My Moments [Nm]"
  Bus Selector2/1 -> SIDE SLIP ANGLE CALCULATION/1(Vx [m/s])  "<Vx [m/s]>"
  Bus Selector2/2 -> SIDE SLIP ANGLE CALCULATION/2(Vy [m/s])  "<Vy [m/s]>"
  Bus Selector2/3 -> TIRE VELOCITIES/7(psidot)  "<psi_dot [rad/s]>"
  Bus Selector5/1 -> TIRE FORCES AND WHEEL DYNAMICS/21(TFL)  "<TFL [Nm]>"
  Bus Selector5/2 -> TIRE FORCES AND WHEEL DYNAMICS/22(TFR)  "<TFR [Nm]>"
  Bus Selector5/3 -> TIRE FORCES AND WHEEL DYNAMICS/23(TRL)  "<TRL [Nm]>"
  Bus Selector5/4 -> TIRE FORCES AND WHEEL DYNAMICS/24(TRR)  "<TRR [Nm]>"

== system VDSE_2019b1/14-DOF VEHICLE MODEL/EQUATIONS OF MOTION FOR CHASSIS/Pitch Dynamics/Downforce ==
  Vx : Inport
  Gain : Gain  Gain=-0.5*rho*clF*A
  Gain{1,3,5,7} (4 alike) : Gain  Gain=0.5
  Gain2 : Gain  Gain=-0.5*rho*clF*A
  Gain4 : Gain  Gain=-0.5*rho*clR*A
  Gain6 : Gain  Gain=-0.5*rho*clR*A
  Square{,1..3} (4 alike) : Math  Operator=square
  fFLz_overall : Outport
  fFRz_overall : Outport  Port=2
  fRLz_overall : Outport  Port=3
  fRRz_overall : Outport  Port=4
  wires:
  Gain/1 -> Gain1/1
  Square/1 -> Gain/1
  Gain1/1 -> fFLz_overall/1
  Square1/1 -> Gain2/1
  Gain2/1 -> Gain3/1
  Gain3/1 -> fFRz_overall/1
  Vx/1 -> Square/1, Square1/1, Square2/1, Square3/1
  Gain6/1 -> Gain7/1
  Square3/1 -> Gain6/1
  Square2/1 -> Gain4/1
  Gain4/1 -> Gain5/1
  Gain5/1 -> fRLz_overall/1
  Gain7/1 -> fRRz_overall/1

== system VDSE_2019b1/14-DOF VEHICLE MODEL/EQUATIONS OF MOTION FOR CHASSIS/Roll Dynamics/Downforce ==
  Vx : Inport
  Gain : Gain  Gain=-0.5*rho*clF*A
  Gain{1,3,5,7} (4 alike) : Gain  Gain=0.5
  Gain2 : Gain  Gain=-0.5*rho*clF*A
  Gain4 : Gain  Gain=-0.5*rho*clR*A
  Gain6 : Gain  Gain=-0.5*rho*clR*A
  Square{,1..3} (4 alike) : Math  Operator=square
  fFLz_overall : Outport
  fFRz_overall : Outport  Port=2
  fRLz_overall : Outport  Port=3
  fRRz_overall : Outport  Port=4
  wires:
  Gain/1 -> Gain1/1
  Square/1 -> Gain/1
  Gain1/1 -> fFLz_overall/1
  Square1/1 -> Gain2/1
  Gain2/1 -> Gain3/1
  Gain3/1 -> fFRz_overall/1
  Vx/1 -> Square/1, Square1/1, Square2/1, Square3/1
  Gain6/1 -> Gain7/1
  Square3/1 -> Gain6/1
  Square2/1 -> Gain4/1
  Gain4/1 -> Gain5/1
  Gain5/1 -> fRLz_overall/1
  Gain7/1 -> fRRz_overall/1

== system VDSE_2019b1/14-DOF VEHICLE MODEL/EQUATIONS OF MOTION FOR CHASSIS/Vertical Dynamics/Downforce ==
  Vx : Inport
  Gain : Gain  Gain=-0.5*rho*clF*A
  Gain{1,3,5,7} (4 alike) : Gain  Gain=0.5
  Gain2 : Gain  Gain=-0.5*rho*clF*A
  Gain4 : Gain  Gain=-0.5*rho*clR*A
  Gain6 : Gain  Gain=-0.5*rho*clR*A
  Square{,1..3} (4 alike) : Math  Operator=square
  fFLz_overall : Outport
  fFRz_overall : Outport  Port=2
  fRLz_overall : Outport  Port=3
  fRRz_overall : Outport  Port=4
  wires:
  Gain/1 -> Gain1/1
  Square/1 -> Gain/1
  Gain1/1 -> fFLz_overall/1
  Square1/1 -> Gain2/1
  Gain2/1 -> Gain3/1
  Gain3/1 -> fFRz_overall/1
  Vx/1 -> Square/1, Square1/1, Square2/1, Square3/1
  Gain6/1 -> Gain7/1
  Square3/1 -> Gain6/1
  Square2/1 -> Gain4/1
  Gain4/1 -> Gain5/1
  Gain5/1 -> fRLz_overall/1
  Gain7/1 -> fRRz_overall/1

== system VDSE_2019b1/14-DOF VEHICLE MODEL/POWERTRAIN AND BRAKES/4 Wheels Drive_3 Motors Powertrain/Subsystem1 ==
  Engine rpm : Inport
  1-D Lookup Table : Lookup_n-D  NumberOfTableDimensions=1  BreakpointsForDimension1=Gear_numbers  Table=GR  ExtrapMethod=Clip  InternalRulePriority=Speed  RndMeth=Simplest
  Constant : Constant  Value=initial_gear
  Constant1 : Constant  Value=enableDriverControl
  Constant2 : Constant  Value=minrpm
  Constant3 : Constant  Value=maxrpm
  Delay : Delay  DelayLength=1  InitialCondition=initial_gear
  Delay1 : Delay  DelayLength=1  InitialCondition=800
  MATLAB Function : MATLAB Function  TreatAsAtomicUnit=on
  Switch : Switch  Criteria=u2 > Threshold  SaturateOnIntegerOverflow=off  InputSameDT=off
  Gear No. : Outport
  Gear_Ratio : Outport  Port=2
  wires:
  Delay1/1 -> MATLAB Function/1(rpm)
  Constant2/1 -> MATLAB Function/3(minrpm)
  Delay/1 -> MATLAB Function/2(gr_no_previous)
  Constant1/1 -> Switch/2
  1-D Lookup Table/1 -> Gear_Ratio/1  "Gear_Ratio"
  MATLAB Function/1(gr_no) -> Gear No./1, Switch/1, Delay/1  "Gear No."
  Constant/1 -> Switch/3
  Switch/1 -> 1-D Lookup Table/1
  Constant3/1 -> MATLAB Function/4(maxrpm)
  Engine rpm/1 -> Delay1/1

== system VDSE_2019b1/14-DOF VEHICLE MODEL/POWERTRAIN AND BRAKES/VCU/Subsystem1 ==
  TrqRequst_Act_Nm : Inport
  VehSpd_kph : Inport  Port=2
  OmegaRL : Inport  Port=3
  OmegaRR : Inport  Port=4
  Add : Sum
  Function-Call Generator : simulink/Ports & Subsystems/Function-Call Generator  sample_time=0.01  numberOfIterations=1  DisallowWideOutput=off
  Gain : Gain  Gain=1/2
  Gain1 : Gain  Gain=rR*180/pi
  Manual Switch : ManualSwitch
  Subsystem : Subsystem
  mps2kph : Gain  Gain=3.6
  TCS_flgActv : Outport
  TCS_TrqRequestFinal_Nm : Outport  Port=2
  wires:
  TrqRequst_Act_Nm/1 -> Manual Switch/2, Subsystem/2(TrqRequst_Act_Nm)
  VehSpd_kph/1 -> Subsystem/3(VehSpd_kph)
  Manual Switch/1 -> TCS_TrqRequestFinal_Nm/1
  Gain/1 -> mps2kph/1
  OmegaRR/1 -> Add/2
  OmegaRL/1 -> Add/1
  Function-Call Generator/1 -> Subsystem/Trigger
  Subsystem/1(TCS_flgActv) -> TCS_flgActv/1  "TCS_flgActv"
  Add/1 -> Gain1/1
  mps2kph/1 -> Subsystem/1(WhlSpd_kph)  "VehSpd_kph"
  Subsystem/2(TCS_TrqRequestFinal_Nm) -> Manual Switch/1
  Gain1/1 -> Gain/1

== system VDSE_2019b1/14-DOF VEHICLE MODEL/POWERTRAIN AND BRAKES/VCU/坐标系转换 ==
  note: cos模块的单位是弧度制、
  note: 未考虑漂移工况
  note: 顺时针为正，逆时针为负。
  WhlSpdFL_mps : Inport
  WhlSpdFR_mps : Inport  Port=2
  WhlSpdRL_mps : Inport  Port=3
  WhlSpdRR_mps : Inport  Port=4
  IMU_YawRate_dps : Inport  Port=5
  WhlStrAngL_deg : Inport  Port=6
  WhlStrAngR_deg : Inport  Port=7
  Add : Sum  Inputs=+-
  Add1 : Sum
  Add2 : Sum  Inputs=+-
  Add3 : Sum
  Asin : Trigonometry  Operator=cos
  Asin1 : Trigonometry  Operator=cos
  Bus Creator : BusCreator  Inputs=4
  Constant : Constant  Value=Ldwr
  Constant1 : Constant  Value=Ldwf
  Gain : Gain  Gain=1/2
  Gain1 : Gain  Gain=1/2
  Gain2 : Gain  Gain=pi/180
  Gain3 : Gain  Gain=pi/180
  Gain4 : Gain  Gain=pi/180
  Product{,1..3} (4 alike) : Product
  Vxii_mps : Outport
  IMU_YawRate_dps1 : Outport  Port=2
  wires:
  Constant/1 -> Gain/1
  Gain/1 -> Product/2
  IMU_YawRate_dps/1 -> Gain4/1  "IMU_YawRate_dps"
  WhlSpdRL_mps/1 -> Add/1  "WhlSpdRL_mps"
  WhlSpdRR_mps/1 -> Add1/2  "WhlSpdRR_mps"
  Product/1 -> [Vldwr]
  [Vldwr] -> Add/2, Add1/1
  WhlSpdFL_mps/1 -> Product1/1  "WhlSpdFL_mps"
  WhlSpdFR_mps/1 -> Product2/2  "WhlSpdFR_mps"
  Constant1/1 -> Gain1/1
  Gain1/1 -> Product3/1
  Product3/1 -> [Vldwf]
  Product1/1 -> Add2/1  "1"
  [Vldwf] -> Add2/2, Add3/1  "3"
  Product2/1 -> Add3/2
  Add2/1 -> Bus Creator/1  "VxFL_mps"
  Add/1 -> Bus Creator/3  "VxRL_mps"
  Add3/1 -> Bus Creator/2  "VxFR_mps"
  Add1/1 -> Bus Creator/4  "VxRR_mps"
  Bus Creator/1 -> Vxii_mps/1
  Asin1/1 -> Product2/1
  WhlStrAngR_deg/1 -> Gain3/1  "WhlStrAngR_deg"
  WhlStrAngL_deg/1 -> Gain2/1  "WhlStrAngL_deg"
  Asin/1 -> Product1/2  "a"
  Gain2/1 -> Asin/1
  Gain3/1 -> Asin1/1
  Gain4/1 -> IMU_YawRate_dps1/1, Product/1, Product3/2

== system VDSE_2019b1/14-DOF VEHICLE MODEL/POWERTRAIN AND BRAKES/VCU/打滑判断 ==
  note: 实践中很难同时满足这三个条件。
      | 一般只满足后两个其中一个即可。
  note: 更改记录：1、理了信号线，更整齐。
      | 2、加速度差，加速度差的微分的判断加入滤波模块。
      | 3、轮速选取改为选取最大轮速。
  note: 选取一个最大轮速
  Vxii_mps : Inport
  IMU_YawRate_dps : Inport  Port=2
  IMU_Aa_mpss : Inport  Port=3
  VehSpdEstiZ1_mps : Inport  Port=4
  Bus Selector : BusSelector  OutputSignals=VxFL_mps,VxFR_mps,VxRL_mps,VxRR_mps
  Cast To Double{,1..3} (4 alike) : DataTypeConversion  OutDataTypeStr=boolean  SaturateOnIntegerOverflow=off  RndMeth=Floor
  Logical Operator : Logic  Operator=OR  AllPortsSameDT=off  OutDataTypeStr=boolean
  Logical Operator1 : Logic  AllPortsSameDT=off  OutDataTypeStr=boolean
  Min1 : MinMax  Function=max  Inputs=4
  Mux : Mux
  Mux1 : Mux
  Mux2 : Mux
  Selector : Selector  InputPortWidth=4  IndexOptions=Index vector (dialog)  Indices=[1]  OutputSizes=1
  Selector1 : Selector  InputPortWidth=4  IndexOptions=Index vector (dialog)  Indices=[2]  OutputSizes=1
  Selector2 : Selector  InputPortWidth=4  IndexOptions=Index vector (dialog)  Indices=[3]  OutputSizes=1
  Selector3 : Selector  InputPortWidth=4  IndexOptions=Index vector (dialog)  Indices=[4]  OutputSizes=1
  Terminator : Terminator
  加速度差判断 : Subsystem
  加速度差的微分的判断 : Subsystem
  速差判断 : Subsystem
  WhlSlipFLValid_flag : Outport
  WhlSlipFRValid_flag : Outport  Port=2
  WhlSlipRLValid_flag : Outport  Port=3
  WhlSlipRRValid_flag : Outport  Port=4
  WhlSpdMax_mps : Outport  Port=5
  wires:
  Selector3/1 -> Cast To Double3/1
  Selector2/1 -> Cast To Double2/1
  [IMU_Aa_mpsss] -> 加速度差的微分的判断/5(IMU_Ax_mpss)
  [VehSpdEstiZ1_mps] -> 速差判断/5(VehSpd_mps)
  Bus Selector/3 -> 加速度差的微分的判断/3(<VxRL_mps>), 速差判断/3(<VxRL_mps>), Min1/3, 加速度差判断/3(<VxRL_mps>)  "<VxRL_mps>"
  Selector1/1 -> Cast To Double1/1
  [IMU_Aa_mpsss] -> 加速度差判断/5(IMU_Ax_mpss)
  Bus Selector/4 -> 加速度差判断/4(<VxRR_mps>), Min1/4, 速差判断/4(<VxRR_mps>), 加速度差的微分的判断/4(<VxRR_mps>)  "<VxRR_mps>"
  IMU_YawRate_dps/1 -> [IMU_YawRate_dps]
  Vxii_mps/1 -> Bus Selector/1
  Bus Selector/1 -> 加速度差的微分的判断/1(<VxFL_mps>), 加速度差判断/1(<VxFL_mps>), 速差判断/1(<VxFL_mps>), Min1/1  "<VxFL_mps>"
  VehSpdEstiZ1_mps/1 -> [VehSpdEstiZ1_mps]
  Selector/1 -> Cast To Double/1
  Bus Selector/2 -> 加速度差的微分的判断/2(<VxFR_mps>), 加速度差判断/2(<VxFR_mps>), 速差判断/2(<VxFR_mps>), Min1/2  "<VxFR_mps>"
  IMU_Aa_mpss/1 -> [IMU_Aa_mpsss]
  [IMU_YawRate_dps] -> Terminator/1
  Cast To Double/1 -> WhlSlipFLValid_flag/1  "WhlSlipFLValid_flag"
  Cast To Double1/1 -> WhlSlipFRValid_flag/1  "WhlSlipFRValid_flag"
  Cast To Double2/1 -> WhlSlipRLValid_flag/1  "WhlSlipRLValid_flag"
  Cast To Double3/1 -> WhlSlipRRValid_flag/1  "WhlSlipRRValid_flag"
  速差判断/1(y) -> Mux/1  "速差"
  速差判断/2(y1) -> Mux/2
  速差判断/3(y2) -> Mux/3
  速差判断/4(y3) -> Mux/4
  加速度差判断/1(y) -> Mux1/1  "加速度差"
  加速度差判断/2(y1) -> Mux1/2
  加速度差判断/3(y2) -> Mux1/3
  加速度差判断/4(y3) -> Mux1/4
  加速度差的微分的判断/1(y) -> Mux2/1  "加速度差的微分"
  加速度差的微分的判断/2(y1) -> Mux2/2
  加速度差的微分的判断/3(y2) -> Mux2/3
  加速度差的微分的判断/4(y3) -> Mux2/4
  Mux1/1 -> Logical Operator/1
  Mux2/1 -> Logical Operator/2
  Mux/1 -> Logical Operator1/1
  Logical Operator/1 -> Logical Operator1/2
  Logical Operator1/1 -> Selector3/1, Selector2/1, Selector1/1, Selector/1
  Min1/1 -> WhlSpdMax_mps/1

== system VDSE_2019b1/14-DOF VEHICLE MODEL/POWERTRAIN AND BRAKES/VCU/积分判断 ==
  note: 对加速度进行积分
  note: 计时器，当积分速度大于轮速一个时间后，退出积分速度。
  note: 积分开始时，需要给初始值
  WhlSlipFL_flag : Inport
  WhlSlipFR_flag : Inport  Port=2
  WhlSlipRL_flag : Inport  Port=3
  WhlSlipRR_flag : Inport  Port=4
  IMU_Ax_mpss : Inport  Port=5
  FFVehVxEst_mps : Inport  Port=6
  TrqReq_Nm : Inport  Port=7
  WhlSpdMax_mps : Inport  Port=8
  Add{,3..4,10} (4 alike) : Sum
  Add1 : Sum  Inputs=-+
  Add2 : Sum  Inputs=+-
  Cast To Double : DataTypeConversion  OutDataTypeStr=single  SaturateOnIntegerOverflow=off  RndMeth=Floor
  Cast To Double1 : DataTypeConversion  OutDataTypeStr=boolean  SaturateOnIntegerOverflow=off  RndMeth=Floor
  Compare To Constant : simulink/Logic and Bit Operations/Compare To Constant  relop=>  const=TrqRquRate  OutDataTypeStr=boolean
  Compare To Constant1 : simulink/Logic and Bit Operations/Compare To Constant  relop=<=  const=0  OutDataTypeStr=boolean
  Constant : Constant  Value=single(0)
  InitZORE : Constant  Value=single(0)
  Logical Operator : Logic  Operator=OR  Inputs=4  AllPortsSameDT=off  OutDataTypeStr=boolean
  Logical Operator1 : Logic  Operator=NOT  AllPortsSameDT=off  OutDataTypeStr=boolean
  Logical Operator2 : Logic  Operator=OR  AllPortsSameDT=off  OutDataTypeStr=boolean
  Logical Operator3 : Logic  Operator=NOT  AllPortsSameDT=off  OutDataTypeStr=boolean
  Min : MinMax  Inputs=2
  Product : Product
  Relational Operator9 : RelationalOperator  OutDataTypeStr=boolean  RndMeth=Simplest  InputSameDT=off
  Reset : Constant  Value=single(0)
  ResetDelay : Constant  Value=single(0.1)
  Saturation : Saturate  UpperLimit=200  LowerLimit=-10
  Saturation1 : Saturate  UpperLimit=200  LowerLimit=-10
  Steptime : Constant  Value=single(0.01)
  Switch{1,3..4,6} (4 alike) : Switch  Criteria=u2 ~= 0  SaturateOnIntegerOverflow=off  InputSameDT=off
  Unit Delay{,1..4} (5 alike) : UnitDelay  SampleTime=-1  HasFrameUpgradeWarning=on
  steptime1 : Constant  Value=single(0.01)
  steptime2 : Constant  Value=single(0)
  VxIMU_est : Outport
  IMUVehSpdEstiExit : Outport  Port=2
  wires:
  WhlSlipFL_flag/1 -> Logical Operator/1
  WhlSlipFR_flag/1 -> Logical Operator/2
  WhlSlipRL_flag/1 -> Logical Operator/3
  WhlSlipRR_flag/1 -> Logical Operator/4
  Logical Operator/1 -> Logical Operator1/1
  Unit Delay/1 -> Saturation1/1
  Add/1 -> Switch1/1
  Constant/1 -> Switch1/3
  Logical Operator1/1 -> Logical Operator2/1
  TrqReq_Nm/1 -> Cast To Double/1
  Unit Delay4/1 -> Add1/1
  Add1/1 -> Compare To Constant/1
  Compare To Constant/1 -> Logical Operator2/2
  [IMUAccIns_ACT] -> Switch1/2
  Logical Operator2/1 -> Cast To Double1/1
  Add2/1 -> Compare To Constant1/1
  WhlSpdMax_mps/1 -> Add2/1
  Saturation1/1 -> Add/2
  Product/1 -> Add/1
  IMU_Ax_mpss/1 -> Product/1
  steptime1/1 -> Product/2
  Saturation/1 -> Add3/1
  Add3/1 -> Add2/2, VxIMU_est/1  "VxIMU_est"
  Switch6/1 -> Min/1
  ResetDelay/1 -> Relational Operator9/2, Min/2
  Compare To Constant1/1 -> Switch6/2
  Add10/1 -> Switch6/1
  Steptime/1 -> Add10/2
  Min/1 -> Relational Operator9/1, Unit Delay2/1
  Reset/1 -> Switch6/3
  Unit Delay2/1 -> Add10/1
  Unit Delay3/1 -> Logical Operator3/1
  InitZORE/1 -> Switch4/3
  Logical Operator3/1 -> Switch3/2
  Switch3/1 -> Add3/2, Unit Delay1/1  "VehSpdInit_mps"
  Switch4/1 -> Switch3/1
  Cast To Double/1 -> Unit Delay4/1, Add1/2
  [IMUAccIns_ACT] -> Unit Delay3/1, Switch4/2  "IMUAccIns_ACT"
  Relational Operator9/1 -> IMUVehSpdEstiExit/1  "IMUVehSpdEstiExit"
  Cast To Double1/1 -> [IMUAccIns_ACT]
  Unit Delay1/1 -> Switch3/3
  Add4/1 -> Switch4/1
  FFVehVxEst_mps/1 -> Add4/2
  steptime2/1 -> Add4/1
  Switch1/1 -> Saturation/1, Unit Delay/1

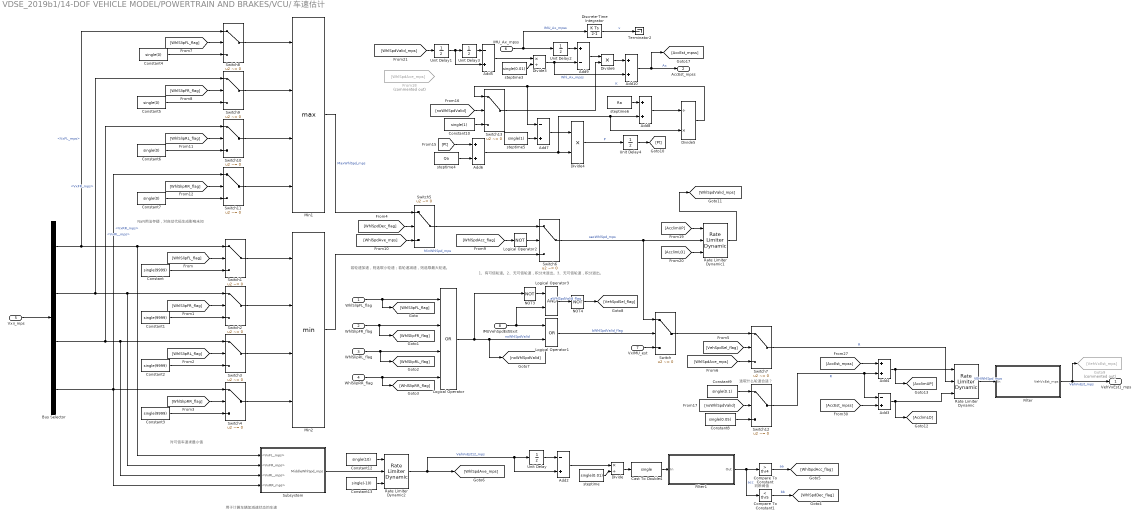
== system VDSE_2019b1/14-DOF VEHICLE MODEL/POWERTRAIN AND BRAKES/VCU/车速估计 ==
  note: 用于计算车辆加减速状态的车速
  note: 1、有可信轮速。2、无可信轮速，积分未退出。3、无可信轮速，积分退出。
  note: 选取什么轮速合适？
  note: 判断阈值
  note: 若轮速加速，则选取小轮速；若轮速减速，则选取最大轮速。
  note: NaN用法存疑，对自动代码生成影响未知
  note: 对可信车速求最小值
  WhlSlipFL_flag : Inport
  WhlSlipFR_flag : Inport  Port=2
  WhlSlipRL_flag : Inport  Port=3
  WhlSlipRR_flag : Inport  Port=4
  Vxii_mps : Inport  Port=5
  IMU_Ax_mpss : Inport  Port=6
  VxIMU_est : Inport  Port=7
  IMUVehSpdEstiExit : Inport  Port=8
  Add{4,6,8,10} (4 alike) : Sum
  Add{2..3,5,7} (4 alike) : Sum  Inputs=-+
  Add9 : Sum  Inputs=+-
  Bus Selector : BusSelector  OutputSignals=VxFL_mps,VxFR_mps,VxRL_mps,VxRR_mps
  Cast To Double4 : DataTypeConversion  OutDataTypeStr=single  SaturateOnIntegerOverflow=off  RndMeth=Floor
  Compare To Constant : simulink/Logic and Bit Operations/Compare To Constant  relop=>  const=thr4  OutDataTypeStr=boolean
  Compare To Constant1 : simulink/Logic and Bit Operations/Compare To Constant  relop=<  const=thr5  OutDataTypeStr=boolean
  Constant{,1..3} (4 alike) : Constant  Value=single(9999)
  Constant10 : Constant  Value=single(1)
  Constant12 : Constant  Value=single(10)
  Constant13 : Constant  Value=single(-10)
  Constant{4..7} (4 alike) : Constant  Value=single(0)
  Constant8 : Constant  Value=single(0.05)
  Constant9 : Constant  Value=single(0.1)
  Discrete-Time Integrator : DiscreteIntegrator  SampleTime=-1  ICPrevOutput=DiscIntNeverNeededParam  ICPrevScaledInput=DiscIntNeverNeededParam
  Divide : Product  Inputs=*/
  Divide3 : Product  Inputs=*/
  Divide4 : Product  Inputs=**
  Divide5 : Product  Inputs=/*
  Divide6 : Product  Inputs=**
  Filter : Subsystem
  Filter1 : Subsystem
  From18 : From  Commented=on  GotoTag=WhlSpdAve_mps
  Goto9 : Goto  Commented=on  GotoTag=VehVxEst_mps
  Logical Operator : Logic  Operator=OR  Inputs=4  AllPortsSameDT=off  OutDataTypeStr=boolean
  Logical Operator1 : Logic  Operator=OR  AllPortsSameDT=off  OutDataTypeStr=boolean
  Logical Operator2 : Logic  Operator=NOT  AllPortsSameDT=off  OutDataTypeStr=boolean
  Logical Operator3 : Logic  AllPortsSameDT=off  OutDataTypeStr=boolean
  Min1 : MinMax  Function=max  Inputs=4
  Min2 : MinMax  Inputs=4
  NOT3 : Logic  Operator=NOT  AllPortsSameDT=off  OutDataTypeStr=boolean
  NOT4 : Logic  Operator=NOT  AllPortsSameDT=off  OutDataTypeStr=boolean
  Rate Limiter Dynamic : simulink/Discontinuities/Rate Limiter Dynamic
  Rate Limiter Dynamic1 : simulink/Discontinuities/Rate Limiter Dynamic
  Rate Limiter Dynamic2 : simulink/Discontinuities/Rate Limiter Dynamic
  Subsystem : Subsystem
  Switch{,1..13} (14 alike) : Switch  Criteria=u2 ~= 0  SaturateOnIntegerOverflow=off  InputSameDT=off
  Terminator2 : Terminator
  Unit Delay{,1..3} (4 alike) : UnitDelay  SampleTime=-1  HasFrameUpgradeWarning=on
  Unit Delay4 : UnitDelay  InitialCondition=0.01  SampleTime=-1  HasFrameUpgradeWarning=on
  steptime : Constant  Value=single(0.01)
  steptime3 : Constant  Value=single(0.01)
  steptime4 : Constant  Value=Qa
  steptime5 : Constant  Value=single(1)
  steptime6 : Constant  Value=Ra
  VehVxEst1_mps : Outport
  AccEst_mpss : Outport  Port=2
  wires:
  Compare To Constant/1 -> [WhlSpdAcc_flag]  "aa"
  Vxii_mps/1 -> Bus Selector/1
  WhlSlipRR_flag/1 -> [WhlSlipRR_flag], Logical Operator/4
  Logical Operator3/1 -> NOT4/1  "aWhlSpdValid_flag"
  [VehSpdSel_flag] -> Switch7/2
  Logical Operator2/1 -> Switch6/2
  [WhlSlipFL_flag] -> Switch1/2
  Switch5/1 -> Switch6/1
  Constant/1 -> Switch1/3
  Compare To Constant1/1 -> [WhlSpdDec_flag]  "bb"
  Unit Delay/1 -> Add2/1
  [WhlSpdAve_mps] -> Switch5/3
  Filter1/1(Out) -> Compare To Constant1/1, Compare To Constant/1  "acc"
  Constant3/1 -> Switch4/3
  Logical Operator1/1 -> Switch/2  "bWhlSpdValid_flag"
  Switch4/1 -> Min2/4
  Constant2/1 -> Switch3/3
  [WhlSlipRR_flag] -> Switch4/2
  Switch1/1 -> Min2/1
  WhlSlipFR_flag/1 -> [WhlSlipFR_flag], Logical Operator/2
  [WhlSpdAcc_flag] -> Logical Operator2/1
  [WhlSlipRL_flag] -> Switch3/2
  Switch2/1 -> Min2/2
  Logical Operator/1 -> [noWhlSpdValid], Logical Operator1/2, NOT3/1  "noWhlSpdValid"
  WhlSlipFL_flag/1 -> [WhlSlipFL_flag], Logical Operator/1
  Constant1/1 -> Switch2/3
  Cast To Double4/1 -> Filter1/1(In)
  [WhlSpdDec_flag] -> Switch5/2
  [WhlSlipFR_flag] -> Switch2/2
  WhlSlipRL_flag/1 -> [WhlSlipRL_flag], Logical Operator/3
  Switch3/1 -> Min2/3
  [WhlSpdAve_mps] -> Switch7/3
  Add2/1 -> Divide/1
  Divide/1 -> Cast To Double4/1
  steptime/1 -> Divide/2
  Bus Selector/1 -> Switch8/1, Subsystem/1(<VxFL_mps>), Switch1/1  "<VxFL_mps>"
  Bus Selector/4 -> Subsystem/4(<VxRR_mps>), Switch11/1, Switch4/1  "<VxRR_mps>"
  [WhlSlipFR_flag] -> Switch9/2
  Bus Selector/2 -> Switch9/1, Subsystem/2(<VxFR_mps>), Switch2/1  "<VxFR_mps>"
  Constant5/1 -> Switch9/3
  Bus Selector/3 -> Switch10/1, Subsystem/3(<VxRL_mps>), Switch3/1  "<VxRL_mps>"
  [WhlSlipRL_flag] -> Switch10/2
  [WhlSlipRR_flag] -> Switch11/2
  Constant6/1 -> Switch10/3
  Constant7/1 -> Switch11/3
  Constant4/1 -> Switch8/3
  [WhlSlipFL_flag] -> Switch8/2
  Switch8/1 -> Min1/1
  Switch9/1 -> Min1/2
  Switch10/1 -> Min1/3
  Switch11/1 -> Min1/4
  Min1/1 -> Switch5/1  "MaxWhlSpd_mps"
  Subsystem/1(MiddleWhlSpd_mps) -> Rate Limiter Dynamic2/2
  Constant12/1 -> Rate Limiter Dynamic2/1
  Constant13/1 -> Rate Limiter Dynamic2/3
  Rate Limiter Dynamic2/1 -> [WhlSpdAve_mps], Add2/2, Unit Delay/1  "VehVxEst12_mps"
  Min2/1 -> Switch6/3  "MinWhlSpd_mps"
  IMUVehSpdEstiExit/1 -> Logical Operator3/2, Logical Operator1/1
  NOT3/1 -> Logical Operator3/1
  NOT4/1 -> [VehSpdSel_flag]
  Divide5/1 -> Add7/1, Switch13/1  "K"
  Unit Delay3/1 -> Add5/1
  steptime3/1 -> Divide3/2
  Add5/1 -> Divide3/1
  Unit Delay4/1 -> [Pt]
  [Pt] -> Add6/1
  steptime4/1 -> Add6/2
  Add6/1 -> Divide5/2, Add8/2, Divide4/2
  steptime5/1 -> Add7/2
  Add7/1 -> Divide4/1
  Divide4/1 -> Unit Delay4/1  "P"
  steptime6/1 -> Add8/1
  Add8/1 -> Divide5/1
  Divide3/1 -> Add10/2, Add9/2  "Whl_Ax_mpss"
  Add9/1 -> Divide6/1
  Divide6/1 -> Add10/1
  Add10/1 -> AccEst_mpss/1, [AccEst_mpss]  "Ax"
  IMU_Ax_mpss/1 -> Unit Delay2/1, Discrete-Time Integrator/1  "IMU_Ax_mpss"
  VxIMU_est/1 -> Switch/3
  Filter/1(VehVxEst_mps) -> VehVxEst1_mps/1, Goto9/1  "VehVxEst_mps"
  Switch/1 -> Switch7/1
  Discrete-Time Integrator/1 -> Terminator2/1  "v"
  [AccEst_mpss] -> Add4/1
  [AccEst_mpss] -> Add3/2
  [WhlSpdValid_mps] -> Unit Delay1/1
  Unit Delay2/1 -> Add9/1
  Switch6/1 -> Switch/1, Rate Limiter Dynamic1/2  "secWhlSpd_mps"
  Add4/1 -> [AcclimUP], Rate Limiter Dynamic/1
  Add3/1 -> [AcclimLO], Rate Limiter Dynamic/3
  Switch7/1 -> Rate Limiter Dynamic/2  "R"
  Rate Limiter Dynamic/1 -> Filter/1(In)  "VEHWhlSpd_mps"
  Rate Limiter Dynamic1/1 -> [WhlSpdValid_mps]
  Unit Delay1/1 -> Add5/2, Unit Delay3/1
  [noWhlSpdValid] -> Switch12/2
  Constant8/1 -> Switch12/3
  Constant9/1 -> Switch12/1
  Switch12/1 -> Add3/1, Add4/2  "R"
  Switch13/1 -> Divide6/2
  [noWhlSpdValid] -> Switch13/2
  Constant10/1 -> Switch13/3
  [AcclimUP] -> Rate Limiter Dynamic1/1
  [AcclimLO] -> Rate Limiter Dynamic1/3
